simulink model "vehicle_motion_model_final_temp"  (R2021b)
settings: Solver=ode5  StartTime=0.0  StopTime=600  FixedStep=0.001  RelTol=1e-3
StopFcn:
  | % stop simulation callback function
  | figure(1);
  | out.x_gt.data = permute(out.x_gt.data,[3, 1, 2]);
  | plot3(out.x_gt.data(:, 1), out.x_gt.data(:, 2), -out.x_gt.data(:, 3), 'Color', 'r', 'LineWidth', 1.5);
  | legend('Истинная траектория')
  | xlabel('X, \itм');
  | ylabel('Y, \itм');
  | zlabel('Z, \itм');
  | figure(2);
  | plot3(out.x.data(:, 1), out.x.data(:, 2), -out.x.data(:, 3), 'Color', 'b', 'LineWidth', 1.5);
  | hold on;
  | xlabel('X, \itм');
  | ylabel('Y, \itм');
  | zlabel('Z, \itм');
  | % legend('pos')
  | hold on;
  | plot3(out.x_gt.data(:, 1), out.x_gt.data(:, 2), -out.x_gt.data(:, 3), 'Color', 'r', 'LineWidth', 1.5);
  | hold on;
  | legend('Рассчитанная траектория', 'Истинная траектория')
  | % errors
  | figure(3);
  | yyaxis left;
  | plot(out.hor_err_fus.time, out.hor_err_fus.data, 'Color', 'b', 'LineWidth', 1.5);
  | xlabel('время, \itс');
  | ylabel('Горизонтальная ошибка, \itм');
  | hold on;
  | yyaxis right;
  | plot(out.ver_err_fus.time, out.ver_err_fus.data, 'Color', 'r', 'LineWidth', 1.5);
  | ylabel('Вертикальная ошибка, \itм');
  | legend('Горизонтальная позиционная ошибка', 'Вертикальная позиционная ошибка');
  | grid on;
  | figure(4);
  | yyaxis left;
  | plot(out.hor_err_ins.time, out.hor_err_ins.data, '-', 'Color', 'b', 'LineWidth', 1.5);
  | xlabel('время, \itс');
  | ylabel('Горизонтальная ошибка, \itм');
  | hold on;
  | yyaxis right;
  | plot(out.ver_err_ins.time, out.ver_err_ins.data, '-', 'Color', 'r', 'LineWidth', 1.5);
  | ylabel('Вертикальная ошибка, \itм');
  | legend('Горизонтальная позиционная ошибка', 'Вертикальная позиционная ошибка');
  | grid on;
model workspace (MAT data in the model file):
  AxlIxx = 62.3745166667
  AxlM = 160
  Cps = 2
  CzWhlAxl = 557955.087061
  DCT_Param : object (value not decoded)
  Downshift_Speeds = [9.5625 12.9375 16.3125 19.6875 23.0625 26.4375 29.8125 33.1875 36.5625 39.9375 43.3125 46.6875 ... (28 elements, 4x7)]
  F0zWhlAxl = 16132.2380068
  HTCH : object (value not decoded)
  Hmax = 0.25
  KzWhlAxl = 58428920.0848
  NCyl = 6
  Pedal_Positions = [0.1 0.4 0.5 0.9]
  Pstd = 101325
  Q = [1  0  0; 0  1  0; 0  0  1]
  Rair = 287
  SUS : object (value not decoded)
  TRA : object (value not decoded)
  Trans : object (value not decoded)
  Tstd = 293.15
  Upshift_Speeds = [12.9375 16.3125 19.6875 33 26.4375 29.8125 33.1875 52.5 39.9375 43.3125 46.6875 77.25 ... (28 elements, 4x7)]
  VEH : object (value not decoded)
  Vd = 0.00346
  WH : Mass (value not decoded)
  dt3D = 0.05
  f_air = [0 0 0 0 0 0 0 0 0 0 0 0 ... (256 elements, 16x16)]
  f_co = [0 0 0 0 0 0 0 0 0 0 0 0 ... (256 elements, 16x16)]
  f_co2 = [0 0 0 0 0 0 0 0 0 0 0 0 ... (256 elements, 16x16)]
  f_eff = [352.135682859 352.135682859 320.724378192 303.655312657 295.930136708 291.240087194 291.240271258 291.240312459 291.240275452 291.240198499 291.240100781 291.240018769 ... (256 elements, 16x16)]
  f_fuel = [0 0 0 0 0 0 0 0 0 0 0 0 ... (256 elements, 16x16)]
  f_hc = [0 0 0 0 0 0 0 0 0 0 0 0 ... (256 elements, 16x16)]
  f_nox = [0 0 0 0 0 0 0 0 0 0 0 0 ... (256 elements, 16x16)]
  f_pm = [0 0 0 0 0 0 0 0 0 0 0 0 ... (256 elements, 16x16)]
  f_susp_axl_bp = [1 2]
  f_susp_dz_bp = [-0.325022776267 -0.315022776267 -0.305022776267 -0.205022776267 -0.105022776267 -0.00502277626717 0.0949772237328 0.194977223733 0.204977223733 0.214977223733]
  f_susp_dzdot_bp = [-3 -0.3 -0.2 -0.1 0 0.1 0.2 0.3 3]
  f_susp_fmz = [-144070.391448 -93629.24037 -75929.1118915 -20630.5828179 -15385.48216 -10140.3815021 -4895.28084414 349.819813785 -31916.3973792 18437.6709544 -83996.1993354 -33555.0482577 ... (43920 elements, 10x9x61x2x4)]
  f_susp_geom = [0 0 0 0 0 0 0 0 0 0 0 0 ... (3660 elements, 10x61x2x3)]
  f_susp_strgdelta_bp = [-0.523598775598 -0.506145483078 -0.488692190558 -0.471238898038 -0.453785605519 -0.436332312999 -0.418879020479 -0.401425727959 -0.383972435439 -0.366519142919 -0.349065850399 -0.331612557879 ... (61 elements, 1x61)]
  f_tbrake = [0 76.8593923996 105.140482948 131.533638111 157.926793274 176.658631717 176.65727296 176.656856686 176.656879077 176.657093756 176.657404516 176.65772406 ... (256 elements, 16x16)]
  f_tbrake_n_bpt = [0 649.519052838 912.419621844 1175.32019085 1438.22075986 1701.12132886 1964.02189787 2226.92246687 2489.82303588 2752.72360489 3015.62417389 3278.5247429 ... (16 elements, 1x16)]
  f_tbrake_t_bpt = [0 34.6410161514 61.0341713143 87.4273264773 113.82048164 140.213636803 166.606791966 192.999947129 219.393102292 245.786257455 272.179412618 298.572567781 ... (16 elements, 1x16)]
  f_texh = [766.752464599 766.752464599 786.17542386 801.679939032 884.591982581 910.574397722 910.571871054 910.570774534 910.570601632 910.570821151 910.571247242 910.571639815 ... (256 elements, 16x16)]
  f_twc_eff_co = [0.17 0.25 0.45 0.99 0.99 0.99 0.99]
  f_twc_eff_hc = [0.21 0.375 0.75 0.98 0.98 0.98 0.98]
  f_twc_eff_lam = [0.909090909 0.944055944 0.979020979 1 1.013986014 1.048951049 1.083916084]
  f_twc_eff_nox = [0.98 0.98 0.98 0.97 0.05 0.02 0]
  h = 0.134
symbols that are objects in the model workspace (value not decoded): VEH
libraries: aerolibcommonsys x8, sharedtransform x8, sharedutil x7, autolibsharedcommon x7, autolibutils x4, vehdynlibtirecommon x3, dspstat3 x2, mspsensorlib x1, aerolibnav x1, shared6dof x1, autolibshared x1, vehdynlibsuspension x1
(part 7 of 9)

== system vehicle_motion_model_final_temp/Two-Axle Vehicle/Wheels and Tires/Wheels and Tires/Tires/MF Tires ==
  DriveTorque : Inport
  Brake Pressure : Inport  Port=2
  r : Inport  Port=3
  Vx : Inport  Port=4
  Vy : Inport  Port=5
  Camber : Inport  Port=6
  Press : Inport  Port=7  Unit=Pa
  lambda : Inport  Port=8  Unit=1
  Gnd : Inport  Port=9
  FzSusp : Inport  Port=10
  Combined Slip Wheel 2DOF : Subsystem  AncestorBlock=vehdynlibtire/Combined Slip Wheel 2DOF  mask(Combined Slip Wheel 2DOF){tireType=Commercial truck 295/75R22.5, BrakeType=Disc, plySteer=off, turnslip=off, mu_static=.3, mu_kinetic=.2, disk_abore=.05, Rm=.177, num_pads=2, drum_abore=0.0508, drum_a=0.123, drum_c=0.212, drum_r=0.15, drum_theta1=0, drum_theta2=126, brake_p_bpt=[1 11.4736842105263 21.9473684210526 32.4210526315789 42.8947368421053 53.3684210526316 63.8421052631579 74.3157894736842 84.7894736842105 95.2631578947368 105.736842105263 116.210526315789 126.684210526316 137.157894736842 147.631578947368 158.105263157895 168.578947368421 179.052631578947 189.526315789474 200], brake_n_bpt=[0 52.6315789473684 105.263157894737 157.894736842105 210.526315789474 263.157894736842 315.789473684211 368.421052631579 421.052631578947 473.684210526316 526.315789473684 578.947368421053 631.578947368421 684.210526315789 736.842105263158 789.473684210526 842.105263157895 894.736842105263 947.368421052632 1000], f_brake_t=[43.4900602404453 42.5056030554862 41.5350898940194 40.5780454442085 39.6340111501808 38.7025443887544 37.7832176914519 36.8756180088306 35.9793460143796 35.0940154454303 34.2192524787115 33.3546951383474 32.4999927342521 31.6548053290159 30.8188032315107 29.991666515561 29.1730845621415 28.362755623661 27.5603864089927 26.765691687993;498.991217495636 487.695866636631 476.560505099801 465.579679307235 454.748127933653 444.060772460445 433.51270824929 423.099196101319 412.81565427025 402.657650900201 392.620896861006 382.701238955775 372.894653477208 363.197240090814 353.605216024701 344.114910546964 334.722759712992 325.425301366216 316.219170376863 307.10109410434;954.492374750826 932.886130217776 911.585920305583 890.581313170261 869.862244717126 849.419000532136 829.242198807128 809.322774193808 789.651962526121 770.221286354971 751.0225412433 732.047782773203 713.289314220164 694.739674852612 676.391628817892 658.238154578366 640.272434863842 622.48784710877 604.877954344734 587.436496520688;1409.99353200602 1378.07639379892 1346.61133551136 1315.58294703329 1284.9763615006 1254.77722860383 1224.97168936497 1195.5463522863 1166.48827078199 1137.78492180974 1109.42418562559 1081.39432659063 1053.68397496312 1026.28210961441 999.178041611083 972.361398609768 945.822110014692 919.550392851325 893.536738312604 867.771898937035;1865.49468926121 1823.26665738007 1781.63675071715 1740.58458089631 1700.09047828407 1660.13545667552 1620.7011799228 1581.76993037878 1543.32457903786 1505.34855726451 1467.82583000789 1430.74087040806 1394.07863570608 1357.82454437621 1321.96445440427 1286.48464264117 1251.37178516554 1216.61293859388 1182.19552228048 1148.10730135338;2320.9958465164 2268.45692096121 2216.66216592293 2165.58621475934 2115.20459506754 2065.49368474721 2016.43067048064 1967.99350847127 1920.16088729373 1872.91219271928 1826.22747439018 1780.08741422549 1734.47329644903 1689.36697913801 1644.75086719747 1600.60788667257 1556.92146031639 1513.67548433643 1470.85430624835 1428.44270376973;2776.49700377159 2713.64718454235 2651.68758112871 2590.58784862237 2530.31871185102 2470.8519128189 2412.16016103848 2354.21708656376 2296.9971955496 2240.47582817405 2184.62911877248 2129.43395804292 2074.86795719199 2020.9094138998 1967.53727999066 1914.73113070398 1862.47113546724 1810.73803007899 1759.51309021622 1708.77810618608;3231.99816102678 3158.8374481235 3086.71299633449 3015.58948248539 2945.43282863449 2876.21014089059 2807.88965159632 2740.44066465625 2673.83350380547 2608.03946362882 2543.03076315477 2478.78050186034 2415.26261793494 2352.4518486616 2290.32369278385 2228.85437473538 2168.02081061809 2107.80057582154 2048.17187418409 1989.11350860242;3687.49931828197 3604.02771170464 3521.73841154027 3440.59111634842 3360.54694541796 3281.56836896228 3203.61914215416 3126.66424274874 3050.66981206134 2975.60309908359 2901.43240753707 2828.12704567777 2755.6572786779 2683.9942834234 2613.11010557704 2542.97761876678 2473.57048576894 2404.8631215641 2336.83065815196 2269.44891101877;4143.00047553716 4049.21797528579 3956.76382674606 3865.59275021144 3775.66106220143 3686.92659703397 3599.34863271199 3512.88782084123 3427.50612031721 3343.16673453836 3259.83405191936 3177.4735894952 3096.05193942085 3015.5367181852 2935.89651837023 2857.10086279818 2779.12016091979 2701.92566730665 2625.48944211983 2549.78431343512;4598.50163279235 4494.40823886693 4391.78924195184 4290.59438407447 4190.77517898491 4092.28482510566 3995.07812326983 3899.11139893372 3804.34242857308 3710.73036999313 3618.23569630166 3526.82013331263 3436.44660016381 3347.079152947 3258.68293116342 3171.22410682959 3084.66983607064 2998.98821304921 2914.1482260877 2830.11971585147;5054.00279004754 4939.59850244808 4826.81465715762 4715.59601793749 4605.88929576838 4497.64305317735 4390.80761382767 4285.3349770262 4181.17873682896 4078.2940054479 3976.63734068395 3876.16667713006 3776.84126090677 3678.62158770879 3581.46934395661 3485.34735086099 ...(+2764 chars)], tireParamSet=vdynPassCar.mat, PRESMAX=1000000, PRESMIN=10000, FZMAX=28000, FZMIN=100, VXLOW=1, KPUMAX=1.5, KPUMIN=-1.5, ALPMAX=1.5, ALPMIN=-1.5, CAMMAX=0.17453, CAMMIN=-0.17453, LONGVL=16.7, FxRelFreqLwrLim=200*pi, FyRelFreqLwrLim=200*pi, MyRelFreqLwrLim=100*pi, omegao=0, br=1e-3, UNLOADED_RADIUS=0.5132, NOMPRES=793000, FNOMIN=14000, WIDTH=0.295, RIM_RADIUS=0.28575, MASS=54.96, IYY=10.664, GRAVITY=-9.81, zo=.015+VEH.InitialVertPosition, zdoto=0, BREFF=8.25094594147963, DREFF=0.260468730454265, FREFF=0.0735298544471851, Q_RE0=1.00866439868088, Q_V1=0.000760413786224011, Q_V2=0.0463384792019201, Q_FZ1=0, Q_FZ2=15.6870832810226, Q_FZ3=0, Q_FCX=0.138643970247602, Q_FCY=0.10843499565426, Q_FCY2=-0.465763352339538, PFZ1=0.69958166705601, VERTICAL_STIFFNESS=207885.061134007, VERTICAL_DAMPING=1000, BOTTOM_OFFST=.01, BOTTOM_STIFF=2e6, LONGITUDINAL_STIFFNESS=388714.175879854, LATERAL_STIFFNESS=157087.404633332, PCFX1=0.18539229191199, PCFX2=0, PCFX3=0, PCFY1=0.163183345037677, PCFY2=0, PCFY3=0.249094918231954, Q_RA1=0.675942571700787, Q_RA2=0.73800463546164, Q_RB1=1.04487486456705, Q_RB2=-1.191763806629, PCX1=1.58523057950359, PDX1=1.0239116238178, PDX2=-0.0842405110022724, PDX3=0, PEX1=0.110312777158455, PEX2=0.313468516038146, PEX3=0, PEX4=0.0016060905760045, PKX1=21.3872544684023, PKX2=14.0006541873175, PKX3=-0.405326109653452, PHX1=0.000212599305364818, PHX2=0.00115950515263055, PVX1=1.59236164471432e-05, PVX2=0.000104321112127671, PPX1=-0.349461321276586, PPX2=0.387840040616429, PPX3=-0.0969947336569324, PPX4=0.0632271859795801, RBX1=12.7633329850276, RBX2=9.5787123658471, RBX3=0, RCX1=1.02796280922059, REX1=-0.45202516851367, REX2=-0.47304886171176, RHX1=0.000233272373115809, QSX1=-0.00788307788961443, QSX2=0.954629515459396, QSX3=0.0155855777667025, QSX4=0.125904607142414, QSX5=1.01110069703963, QSX6=20.1938577118433, QSX7=0.310818120717083, QSX8=-0.0430823751139655, QSX9=0.636494404888216, QSX10=0.142438060591663, QSX11=0.346766530036373, QSX12=0, QSX13=0, QSX14=0, PPMX1=0, PCY1=1.34299950037631, PDY1=0.878267729082195, PDY2=-0.0644597923147385, PDY3=0, PEY1=-0.809776534470972, PEY2=-0.600180598867198, PEY3=0.0991732552633487, PEY4=-6.5577974035573, PEY5=0, PKY1=-15.5714726518315, PKY2=1.73126522291751, PKY3=0.365349873517229, PKY4=1.98176755955416, PKY5=0, PKY6=-0.884005199550313, PKY7=-0.237259727611847, PHY1=-0.00183370557235628, PHY2=0.00346401302716671, PVY1=-0.00675427560163264, PVY2=0.036379218103843, PVY3=-0.163543984089166, PVY4=-0.491003349625726, PPY1=-0.62059646553185, PPY2=-0.0647824842338686, PPY3=-0.164648843290686, PPY4=0.283193909060098, PPY5=0, RBY1=10.7588809173639, RBY2=7.70420065295029, RBY3=3.40283755070691e-06, RBY4=0, RCY1=1.06691874059059, REY1=0.308244924574305, REY2=7.48775032604508e-06, RHY1=0.0118479204960415, RHY2=7.63650177161071e-06, RVY1=0.0560024425050078, RVY2=7.48487127056197e-06, RVY3=0, RVY4=98.4047026517149, RVY5=2.02759273900054, RVY6=15.7623064923347, QSY1=0.00699077564863536, QSY2=0, QSY3=0.00153535478298811, QSY4=8.55710322455322e-05, QSY5=0, QSY6=0, QSY7=0.89443879773793, QSY8=-0.403227641260894, QBZ1=11.666656027484, QBZ2=-1.30355438574485, QBZ3=0, QBZ4=0.177918305399071, QBZ5=-0.162481135068033, QBZ6=0, QBZ9=30.1445534682089, QBZ10=0, QCZ1=1.29026978207574, QDZ1=0.0886972644991399, QDZ2=-0.0058634820161856, QDZ3=0.3805597481383, QDZ4=0, QDZ6=0.00160914918118959, QDZ7=-0.00211036330862154, QDZ8=-0.13921904912557, QDZ9=0.00816585550028243, QDZ10=0, QDZ11=0, QEZ1=-2.19802254534746, QEZ2=1.01850535789165, QEZ3=0, QEZ4=0.278379679112054, QEZ5=-0.548414722765386, QHZ1=0.00148361198869669, QHZ2=0.00202017567585904, QHZ3=0.240316641332066, QHZ4=-0.210114035738085, PPZ1=-0.443927982388615, PPZ2=0, SSZ1=0.00914999585397887, SSZ2=0.0389830656052735, SSZ3=0, SSZ4=0, PDXP1=0.396718274678791, PDXP2=0, PDXP3=0, PKYP1=1.00587060633573, PDYP1=0.40483048923438, PDYP2=0, PDYP3=0, PDYP4=0, PHYP1=0.992731942067188, PHYP2=0.150352945499914, PHYP3=0, PHYP4=-3.98988682633674, PECP1=0.502379254513503, PECP2=0, QDTP1=10.0178654287947, QCRP1=0.200627747200702, QCRP2=0.0995735881599772, QBRP1=0.0997107127960717, QDRP1=1.01432910167423, QDRP2=0, aMode=2}
      mask prompts: tireType "vdynblks:vehdynLatTire:blkPrm_tireType"; BrakeType "vdynblks:vehdynLatTire:blkPrm_BrakeType"; plySteer "vdynblks:vehdynLatTire:blkPrm_plySteer"; turnslip "vdynblks:vehdynLatTire:blkPrm_turnslip"; mu_static "autoblks_shared:autoblkLongitudinalWheel:blkPrm_mu_static"; mu_kinetic "autoblks_shared:autoblkLongitudinalWheel:blkPrm_mu_kinetic"; disk_abore "autoblks_shared:autoblkLongitudinalWheel:blkPrm_disk_abore"; Rm "autoblks_shared:autoblkLongitudinalWheel:blkPrm_Rm"; num_pads "autoblks_shared:autoblkLongitudinalWheel:blkPrm_num_pads"; drum_abore "autoblks_shared:autoblkLongitudinalWheel:blkPrm_drum_abore"; drum_a "autoblks_shared:autoblkLongitudinalWheel:blkPrm_drum_a"; drum_c "autoblks_shared:autoblkLongitudinalWheel:blkPrm_drum_c"; drum_r "autoblks_shared:autoblkLongitudinalWheel:blkPrm_drum_r"; drum_theta1 "autoblks_shared:autoblkLongitudinalWheel:blkPrm_drum_theta1"; drum_theta2 "autoblks_shared:autoblkLongitudinalWheel:blkPrm_drum_theta2"; brake_p_bpt "autoblks_shared:autoblkLongitudinalWheel:blkPrm_brake_p_bpt"; brake_n_bpt "autoblks_shared:autoblkLongitudinalWheel:blkPrm_brake_n_bpt"; f_brake_t "autoblks_shared:autoblkLongitudinalWheel:blkPrm_f_brake_t"; tireParamSet "vdynblks:vehdynLatTire:blkPrm_tireParamSet"; PRESMAX "vdynblks:vehdynLatTire:blkPrm_PRESMAX"; PRESMIN "vdynblks:vehdynLatTire:blkPrm_PRESMIN"; FZMAX "vdynblks:vehdynLatTire:blkPrm_FZMAX"; FZMIN "vdynblks:vehdynLatTire:blkPrm_FZMIN"; VXLOW "vdynblks:vehdynLatTire:blkPrm_VXLOW"; KPUMAX "vdynblks:vehdynLatTire:blkPrm_KPUMAX"; KPUMIN "vdynblks:vehdynLatTire:blkPrm_KPUMIN"; ALPMAX "vdynblks:vehdynLatTire:blkPrm_ALPMAX"; ALPMIN "vdynblks:vehdynLatTire:blkPrm_ALPMIN"; CAMMAX "vdynblks:vehdynLatTire:blkPrm_CAMMAX"; CAMMIN "vdynblks:vehdynLatTire:blkPrm_CAMMIN"; LONGVL "vdynblks:vehdynLatTire:blkPrm_LONGVL"; FxRelFreqLwrLim "Longitudinal relaxation length lower frequency limit, FxRelFreqLwrLim [rad/s]:"; FyRelFreqLwrLim "Lateral relaxation length lower frequency limit, FyRelFreqLwrLim [rad/s]:"; MyRelFreqLwrLim "Rolling relaxation length lower frequency limit, MyRelFreqLwrLim [rad/s]:"; omegao "vdynblks:vehdynLatTire:blkPrm_omegao"; br "vdynblks:vehdynLatTire:blkPrm_br"; UNLOADED_RADIUS "vdynblks:vehdynLatTire:blkPrm_UNLOADED_RADIUS"; NOMPRES "vdynblks:vehdynLatTire:blkPrm_NOMPRES"; FNOMIN "vdynblks:vehdynLatTire:blkPrm_FNOMIN"; WIDTH "vdynblks:vehdynLatTire:blkPrm_WIDTH"; RIM_RADIUS "vdynblks:vehdynLatTire:blkPrm_RIM_RADIUS"; MASS "vdynblks:vehdynLatTire:blkPrm_MASS"; IYY "vdynblks:vehdynLatTire:blkPrm_IYY"; GRAVITY "vdynblks:vehdynLatTire:blkPrm_GRAVITY"; zo "vdynblks:vehdynLatTire:blkPrm_zo"; zdoto "vdynblks:vehdynLatTire:blkPrm_zdoto"; BREFF "vdynblks:vehdynLatTire:blkPrm_BREFF"; DREFF "vdynblks:vehdynLatTire:blkPrm_DREFF"; FREFF "vdynblks:vehdynLatTire:blkPrm_FREFF"; Q_RE0 "vdynblks:vehdynLatTire:blkPrm_Q_RE0"; Q_V1 "vdynblks:vehdynLatTire:blkPrm_Q_V1"; Q_V2 "vdynblks:vehdynLatTire:blkPrm_Q_V2"; Q_FZ1 "vdynblks:vehdynLatTire:blkPrm_Q_FZ1"; Q_FZ2 "vdynblks:vehdynLatTire:blkPrm_Q_FZ2"; Q_FZ3 "vdynblks:vehdynLatTire:blkPrm_Q_FZ3"; Q_FCX "vdynblks:vehdynLatTire:blkPrm_Q_FCX"; Q_FCY "vdynblks:vehdynLatTire:blkPrm_Q_FCY"; Q_FCY2 "vdynblks:vehdynLatTire:blkPrm_Q_FCY2"; PFZ1 "vdynblks:vehdynLatTire:blkPrm_PFZ1"; VERTICAL_STIFFNESS "vdynblks:vehdynLatTire:blkPrm_VERTICAL_STIFFNESS"; VERTICAL_DAMPING "vdynblks:vehdynLatTire:blkPrm_VERTICAL_DAMPING"; BOTTOM_OFFST "vdynblks:vehdynLatTire:blkPrm_BOTTOM_OFFST"; BOTTOM_STIFF "vdynblks:vehdynLatTire:blkPrm_BOTTOM_STIFF"; LONGITUDINAL_STIFFNESS "vdynblks:vehdynLatTire:blkPrm_LONGITUDINAL_STIFFNESS"; LATERAL_STIFFNESS "vdynblks:vehdynLatTire:blkPrm_LATERAL_STIFFNESS"; PCFX1 "vdynblks:vehdynLatTire:blkPrm_PCFX1"; PCFX2 "vdynblks:vehdynLatTire:blkPrm_PCFX2"; PCFX3 "vdynblks:vehdynLatTire:blkPrm_PCFX3"; PCFY1 "vdynblks:vehdynLatTire:blkPrm_PCFY1"; PCFY2 "vdynblks:vehdynLatTire:blkPrm_PCFY2"; PCFY3 "vdynblks:vehdynLatTire:blkPrm_PCFY3"; Q_RA1 "vdynblks:vehdynLatTire:blkPrm_Q_RA1"; Q_RA2 "vdynblks:vehdynLatTire:blkPrm_Q_RA2"; Q_RB1 "vdynblks:vehdynLatTire:blkPrm_Q_RB1"; Q_RB2 "vdynblks:vehdynLatTire:blkPrm_Q_RB2"; PCX1 "vdynblks:vehdynLatTire:blkPrm_PCX1"; PDX1 "vdynblks:vehdynLatTire:blkPrm_PDX1"; PDX2 "vdynblks:vehdynLatTire:blkPrm_PDX2"; PDX3 "vdynblks:vehdynLatTire:blkPrm_PDX3"; PEX1 "vdynblks:vehdynLatTire:blkPrm_PEX1"; PEX2 "vdynblks:vehdynLatTire:blkPrm_PEX2"; PEX3 "vdynblks:vehdynLatTire:blkPrm_PEX3"; PEX4 "vdynblks:vehdynLatTire:blkPrm_PEX4"; PKX1 "vdynblks:vehdynLatTire:blkPrm_PKX1"; PKX2 "vdynblks:vehdynLatTire:blkPrm_PKX2"; PKX3 "vdynblks:vehdynLatTire:blkPrm_PKX3"; PHX1 "vdynblks:vehdynLatTire:blkPrm_PHX1"; PHX2 "vdynblks:vehdynLatTire:blkPrm_PHX2"; PVX1 "vdynblks:vehdynLatTire:blkPrm_PVX1"; PVX2 "vdynblks:vehdynLatTire:blkPrm_PVX2"; PPX1 "vdynblks:vehdynLatTire:blkPrm_PPX1"; PPX2 "vdynblks:vehdynLatTire:blkPrm_PPX2"; PPX3 "vdynblks:vehdynLatTire:blkPrm_PPX3"; PPX4 "vdynblks:vehdynLatTire:blkPrm_PPX4"; RBX1 "vdynblks:vehdynLatTire:blkPrm_RBX1"; RBX2 "vdynblks:vehdynLatTire:blkPrm_RBX2"; RBX3 "vdynblks:vehdynLatTire:blkPrm_RBX3"; RCX1 "vdynblks:vehdynLatTire:blkPrm_RCX1"; REX1 "vdynblks:vehdynLatTire:blkPrm_REX1"; REX2 "vdynblks:vehdynLatTire:blkPrm_REX2"; RHX1 "vdynblks:vehdynLatTire:blkPrm_RHX1"; QSX1 "vdynblks:vehdynLatTire:blkPrm_QSX1"; QSX2 "vdynblks:vehdynLatTire:blkPrm_QSX2"; QSX3 "vdynblks:vehdynLatTire:blkPrm_QSX3"; QSX4 "vdynblks:vehdynLatTire:blkPrm_QSX4"; QSX5 "vdynblks:vehdynLatTire:blkPrm_QSX5"; QSX6 "vdynblks:vehdynLatTire:blkPrm_QSX6"; QSX7 "vdynblks:vehdynLatTire:blkPrm_QSX7"; QSX8 "vdynblks:vehdynLatTire:blkPrm_QSX8"; QSX9 "vdynblks:vehdynLatTire:blkPrm_QSX9"; QSX10 "vdynblks:vehdynLatTire:blkPrm_QSX10"; QSX11 "vdynblks:vehdynLatTire:blkPrm_QSX11"; QSX12 "vdynblks:vehdynLatTire:blkPrm_QSX12"; QSX13 "vdynblks:vehdynLatTire:blkPrm_QSX13"; QSX14 "vdynblks:vehdynLatTire:blkPrm_QSX14"; PPMX1 "vdynblks:vehdynLatTire:blkPrm_PPMX1"; PCY1 "vdynblks:vehdynLatTire:blkPrm_PCY1"; PDY1 "vdynblks:vehdynLatTire:blkPrm_PDY1"; PDY2 "vdynblks:vehdynLatTire:blkPrm_PDY2"; PDY3 "vdynblks:vehdynLatTire:blkPrm_PDY3"; PEY1 "vdynblks:vehdynLatTire:blkPrm_PEY1"; PEY2 "vdynblks:vehdynLatTire:blkPrm_PEY2"; PEY3 "vdynblks:vehdynLatTire:blkPrm_PEY3"; PEY4 "vdynblks:vehdynLatTire:blkPrm_PEY4"; PEY5 "vdynblks:vehdynLatTire:blkPrm_PEY5"; PKY1 "vdynblks:vehdynLatTire:blkPrm_PKY1"; PKY2 "vdynblks:vehdynLatTire:blkPrm_PKY2"; PKY3 "vdynblks:vehdynLatTire:blkPrm_PKY3"; PKY4 "vdynblks:vehdynLatTire:blkPrm_PKY4"; PKY5 "vdynblks:vehdynLatTire:blkPrm_PKY5"; PKY6 "vdynblks:vehdynLatTire:blkPrm_PKY6"; PKY7 "vdynblks:vehdynLatTire:blkPrm_PKY7"; PHY1 "vdynblks:vehdynLatTire:blkPrm_PHY1"; PHY2 "vdynblks:vehdynLatTire:blkPrm_PHY2"; PVY1 "vdynblks:vehdynLatTire:blkPrm_PVY1"; PVY2 "vdynblks:vehdynLatTire:blkPrm_PVY2"; PVY3 "vdynblks:vehdynLatTire:blkPrm_PVY3"; PVY4 "vdynblks:vehdynLatTire:blkPrm_PVY4"; PPY1 "vdynblks:vehdynLatTire:blkPrm_PPY1"; PPY2 "vdynblks:vehdynLatTire:blkPrm_PPY2"; PPY3 "vdynblks:vehdynLatTire:blkPrm_PPY3"; PPY4 "vdynblks:vehdynLatTire:blkPrm_PPY4"; PPY5 "vdynblks:vehdynLatTire:blkPrm_PPY5"; RBY1 "vdynblks:vehdynLatTire:blkPrm_RBY1"; RBY2 "vdynblks:vehdynLatTire:blkPrm_RBY2"; RBY3 "vdynblks:vehdynLatTire:blkPrm_RBY3"; RBY4 "vdynblks:vehdynLatTire:blkPrm_RBY4"; RCY1 "vdynblks:vehdynLatTire:blkPrm_RCY1"; REY1 "vdynblks:vehdynLatTire:blkPrm_REY1"; REY2 "vdynblks:vehdynLatTire:blkPrm_REY2"; RHY1 "vdynblks:vehdynLatTire:blkPrm_RHY1"; RHY2 "vdynblks:vehdynLatTire:blkPrm_RHY2"; RVY1 "vdynblks:vehdynLatTire:blkPrm_RVY1"; RVY2 "vdynblks:vehdynLatTire:blkPrm_RVY2"; RVY3 "vdynblks:vehdynLatTire:blkPrm_RVY3"; RVY4 "vdynblks:vehdynLatTire:blkPrm_RVY4"; RVY5 "vdynblks:vehdynLatTire:blkPrm_RVY5"; RVY6 "vdynblks:vehdynLatTire:blkPrm_RVY6"; QSY1 "vdynblks:vehdynLatTire:blkPrm_QSY1"; QSY2 "vdynblks:vehdynLatTire:blkPrm_QSY2"; QSY3 "vdynblks:vehdynLatTire:blkPrm_QSY3"; QSY4 "vdynblks:vehdynLatTire:blkPrm_QSY4"; QSY5 "vdynblks:vehdynLatTire:blkPrm_QSY5"; QSY6 "vdynblks:vehdynLatTire:blkPrm_QSY6"; QSY7 "vdynblks:vehdynLatTire:blkPrm_QSY7"; QSY8 "vdynblks:vehdynLatTire:blkPrm_QSY8"; QBZ1 "vdynblks:vehdynLatTire:blkPrm_QBZ1"; QBZ2 "vdynblks:vehdynLatTire:blkPrm_QBZ2"; QBZ3 "vdynblks:vehdynLatTire:blkPrm_QBZ3"; QBZ4 "vdynblks:vehdynLatTire:blkPrm_QBZ4"; QBZ5 "vdynblks:vehdynLatTire:blkPrm_QBZ5"; QBZ6 "vdynblks:vehdynLatTire:blkPrm_QBZ6"; QBZ9 "vdynblks:vehdynLatTire:blkPrm_QBZ9"; QBZ10 "vdynblks:vehdynLatTire:blkPrm_QBZ10"; QCZ1 "vdynblks:vehdynLatTire:blkPrm_QCZ1"; QDZ1 "vdynblks:vehdynLatTire:blkPrm_QDZ1"; QDZ2 "vdynblks:vehdynLatTire:blkPrm_QDZ2"; QDZ3 "vdynblks:vehdynLatTire:blkPrm_QDZ3"; QDZ4 "vdynblks:vehdynLatTire:blkPrm_QDZ4"; QDZ6 "vdynblks:vehdynLatTire:blkPrm_QDZ6"; QDZ7 "vdynblks:vehdynLatTire:blkPrm_QDZ7"; QDZ8 "vdynblks:vehdynLatTire:blkPrm_QDZ8"; QDZ9 "vdynblks:vehdynLatTire:blkPrm_QDZ9"; QDZ10 "vdynblks:vehdynLatTire:blkPrm_QDZ10"; QDZ11 "vdynblks:vehdynLatTire:blkPrm_QDZ11"; QEZ1 "vdynblks:vehdynLatTire:blkPrm_QEZ1"; QEZ2 "vdynblks:vehdynLatTire:blkPrm_QEZ2"; QEZ3 "vdynblks:vehdynLatTire:blkPrm_QEZ3"; QEZ4 "vdynblks:vehdynLatTire:blkPrm_QEZ4"; QEZ5 "vdynblks:vehdynLatTire:blkPrm_QEZ5"; QHZ1 "vdynblks:vehdynLatTire:blkPrm_QHZ1"; QHZ2 "vdynblks:vehdynLatTire:blkPrm_QHZ2"; QHZ3 "vdynblks:vehdynLatTire:blkPrm_QHZ3"; QHZ4 "vdynblks:vehdynLatTire:blkPrm_QHZ4"; PPZ1 "vdynblks:vehdynLatTire:blkPrm_PPZ1"; PPZ2 "vdynblks:vehdynLatTire:blkPrm_PPZ2"; SSZ1 "vdynblks:vehdynLatTire:blkPrm_SSZ1"; SSZ2 "vdynblks:vehdynLatTire:blkPrm_SSZ2"; SSZ3 "vdynblks:vehdynLatTire:blkPrm_SSZ3"; SSZ4 "vdynblks:vehdynLatTire:blkPrm_SSZ4"; PDXP1 "vdynblks:vehdynLatTire:blkPrm_PDXP1"; PDXP2 "vdynblks:vehdynLatTire:blkPrm_PDXP2"; PDXP3 "vdynblks:vehdynLatTire:blkPrm_PDXP3"; PKYP1 "vdynblks:vehdynLatTire:blkPrm_PKYP1"; PDYP1 "vdynblks:vehdynLatTire:blkPrm_PDYP1"; PDYP2 "vdynblks:vehdynLatTire:blkPrm_PDYP2"; PDYP3 "vdynblks:vehdynLatTire:blkPrm_PDYP3"; PDYP4 "vdynblks:vehdynLatTire:blkPrm_PDYP4"; PHYP1 "vdynblks:vehdynLatTire:blkPrm_PHYP1"; PHYP2 "vdynblks:vehdynLatTire:blkPrm_PHYP2"; PHYP3 "vdynblks:vehdynLatTire:blkPrm_PHYP3"; PHYP4 "vdynblks:vehdynLatTire:blkPrm_PHYP4"; PECP1 "vdynblks:vehdynLatTire:blkPrm_PECP1"; PECP2 "vdynblks:vehdynLatTire:blkPrm_PECP2"; QDTP1 "vdynblks:vehdynLatTire:blkPrm_QDTP1"; QCRP1 "vdynblks:vehdynLatTire:blkPrm_QCRP1"; QCRP2 "vdynblks:vehdynLatTire:blkPrm_QCRP2"; QBRP1 "vdynblks:vehdynLatTire:blkPrm_QBRP1"; QDRP1 "vdynblks:vehdynLatTire:blkPrm_QDRP1"; QDRP2 "vdynblks:vehdynLatTire:blkPrm_QDRP2"
      mask help: vdynblks:vehdynLatTire:blkDesc
      mask init:
      | vdynMF=vehdynicon('vehdynlibtire',gcb,0);
      mask Help: eval('vdynblkshelp(''vbtireslip'')')
      mask TypeOptions tireType: vdynblks:vehdynLatTire:blkCmb_tireType_c1 | vdynblks:vehdynLatTire:blkCmb_tireType_c2 | vdynblks:vehdynLatTire:blkCmb_tireType_c3 | vdynblks:vehdynLatTire:blkCmb_tireType_c4 | vdynblks:vehdynLatTire:blkCmb_tireType_c5 | vdynblks:vehdynLatTire:blkCmb_tireType_c6 | vdynblks:vehdynLatTire:blkCmb_tireType_c7
      mask Callback tireType: [~]=vehdynicon('vehdynlibtire',gcb,5)
      mask TypeOptions BrakeType: autoblks_shared:autoblkLongitudinalWheel:blkCmb_BrakeType_c1 | autoblks_shared:autoblkLongitudinalWheel:blkCmb_BrakeType_c2 | autoblks_shared:autoblkLongitudinalWheel:blkCmb_BrakeType_c3 | autoblks_shared:autoblkLongitudinalWheel:blkCmb_BrakeType_c4
      mask Callback BrakeType: [~]=vehdynicon('vehdynlibtire',gcb,2)
      mask DialogControl BlockOptions Prompt: autoblks_shared:autoblkLongitudinalWheel:blkDlg_BlockOptions
      mask DialogControl SourceOptions Prompt: vdynblks:vehdynLatTire:blkDlg_SourceOptions
      mask DialogControl tireType Prompt: Tire type:
      mask DialogControl paramOverwrite Prompt: vdynblks:vehdynLatTire:blkPrm_paramOverwrite
      mask DialogControl paramOverwrite Callback: [~]=vehdynicon('vehdynlibtire',gcb,6);
      mask DialogControl BrakeType Prompt: Brake type:
      mask DialogControl plySteer Prompt: Include ply/roll steer behavior
      mask DialogControl turnslip Prompt: Include large turn slip effects
      mask DialogControl WheelParams Prompt: vdynblks:vehdynLatTire:blkDlg_WheelParams
      mask DialogControl brakeParamPanel Prompt: autoblks_shared:autoblkLongitudinalWheel:blkDlg_brakeParamPanel
      mask DialogControl GenParams Prompt: autoblks_shared:autoblkLongitudinalWheel:blkDlg_GenParams
      mask DialogControl mu_static Prompt: Static friction coefficient, mu_static []:
      mask DialogControl mu_kinetic Prompt: Kinetic friction coefficient, mu_kinetic []:
      mask DialogControl DiskBrakeParms Prompt: autoblks_shared:autoblkLongitudinalWheel:blkDlg_DiskBrakeParms
      mask DialogControl disk_abore Prompt: Disc brake actuator bore, disk_abore [m]:
      mask DialogControl Rm Prompt: Brake pad mean radius, Rm [m]:
      mask DialogControl num_pads Prompt: Number of brake pads, num_pads []:
      mask DialogControl DrumBrakeParms Prompt: autoblks_shared:autoblkLongitudinalWheel:blkDlg_DrumBrakeParms
      mask DialogControl drum_abore Prompt: Drum brake actuator bore, drum_abore [m]:
      mask DialogControl drum_a Prompt: Shoe pin to drum center distance, drum_a [m]:
      mask DialogControl drum_c Prompt: Shoe pin center to force application point distance, drum_c [m]:
      mask DialogControl drum_r Prompt: Drum internal radius, drum_r [m]:
      mask DialogControl drum_theta1 Prompt: Shoe pin to pad start angle, drum_theta1 [deg]:
      mask DialogControl drum_theta2 Prompt: Shoe pin to pad end angle, drum_theta2 [deg]:
      mask DialogControl MappedBrakeParms Prompt: autoblks_shared:autoblkLongitudinalWheel:blkDlg_MappedBrakeParms
      mask DialogControl brake_p_bpt Prompt: Brake actuator pressure breakpoints, brake_p_bpt [bar]:
      mask DialogControl brake_n_bpt Prompt: Wheel speed breakpoints, brake_n_bpt [rpm]:
      mask DialogControl f_brake_t Prompt: Brake torque map, f_brake_t [Nm]:
      mask DialogControl PlotBrakeTorqueMap Prompt: autoblks_shared:autoblkLongitudinalWheel:blkDlg_PlotBrakeTorqueMap
      mask DialogControl PlotBrakeTorqueMap Callback: [~]=vehdynicon('vehdynlibtire',gcb,3)
      mask DialogControl tireDataPanel Prompt: vdynblks:vehdynLatTire:blkDlg_tireDataPanel
      mask DialogControl tireParamSet Prompt: Tire file or object, tireParamSet []:
      mask DialogControl getFile Prompt: vdynblks:vehdynLatTire:blkPrm_getFile
      mask DialogControl getFile Callback: [~]=vehdynicon('vehdynlibtire',gcb,4)
      mask DialogControl updateMaskVars Prompt: vdynblks:vehdynLatTire:blkPrm_updateMaskVars
      mask DialogControl updateMaskVars Callback: [~]=vehdynicon('vehdynlibtire',gcb,1)
      mask DialogControl tireParamTab Prompt: vdynblks:vehdynLatTire:blkDlg_tireParamTab
      mask DialogControl simParamPannel Prompt: vdynblks:vehdynLatTire:blkDlg_simParamPannel
      mask DialogControl PRESMAX Prompt: Maximum pressure, PRESMAX [Pa]:
      mask DialogControl PRESMIN Prompt: Minimum pressure, PRESMIN [Pa]:
      mask DialogControl FZMAX Prompt: Maximum normal force, FZMAX [N]:
      mask DialogControl FZMIN Prompt: Minimum normal force, FZMIN [N]:
      mask DialogControl VXLOW Prompt: Velocity tolerance used to handle low velocity situations, VXLOW [m/s]:
      mask DialogControl KPUMAX Prompt: Max allowable slip ratio (absolute), KPUMAX []:
      mask DialogControl KPUMIN Prompt: Minimum allowable slip ratio (absolute), KPUMIN []:
      mask DialogControl ALPMAX Prompt: Max allowable slip angle (absolute), ALPMAX [rad]:
      mask DialogControl ALPMIN Prompt: Minimum allowable slip angle (absolute), ALPMIN [rad]:
      mask DialogControl CAMMAX Prompt: Maximum allowable camber angle, CAMMAX [rad]:
      mask DialogControl CAMMIN Prompt: Minimum allowable camber angle, CAMMIN [rad]:
      mask DialogControl LONGVL Prompt: Nominal longitudinal speed, LONGVL [m/s]:
      mask DialogControl wheelParamPannel Prompt: vdynblks:vehdynLatTire:blkDlg_wheelParamPannel
      mask DialogControl omegao Prompt: Initial rotational velocity, omegao [rad/s]:
      mask DialogControl br Prompt: Rotational damping, br [N*m*s/rad]:
      mask DialogControl UNLOADED_RADIUS Prompt: Unloaded radius, UNLOADED_RADIUS [m]:
      mask DialogControl NOMPRES Prompt: Nominal pressure, NOMPRES [Pa]:
      mask DialogControl FNOMIN Prompt: Nominal normal force, FNOMIN [N]:
      mask DialogControl WIDTH Prompt: Wheel width, WIDTH [m]:
      mask DialogControl RIM_RADIUS Prompt: Rim radius, RIM_RADIUS [m]:
      mask DialogControl inertParamPannel Prompt: vdynblks:vehdynLatTire:blkDlg_inertParamPannel
      mask DialogControl MASS Prompt: Wheel mass, MASS [kg]:
      mask DialogControl IYY Prompt: Rotational inertia (rolling axis), IYY [kg*m^2]:
      mask DialogControl GRAVITY Prompt: Gravity, GRAVITY [m/s^2]:
      mask DialogControl vertParamPannel Prompt: vdynblks:vehdynLatTire:blkDlg_vertParamPannel
      mask DialogControl zo Prompt: Initial tire displacement, zo [m]:
      mask DialogControl zdoto Prompt: Initial wheel vertical velocity (wheel fixed frame), zdoto [m/s]:
      mask DialogControl BREFF Prompt: Effective rolling radius at low load stiffness, BREFF []:
      mask DialogControl DREFF Prompt: Effective rolling radius peak value, DREFF []:
      mask DialogControl FREFF Prompt: Effective rolling radius at high load stiffness, FREFF []:
      mask DialogControl Q_RE0 Prompt: Unloaded to nominal rolling radius ratio, Q_RE0 []:
      mask DialogControl Q_V1 Prompt: Radius rotational speed dependence, Q_V1 []:
      mask DialogControl Q_V2 Prompt: Stiffness rotational speed dependence, Q_V2 []:
      mask DialogControl Q_FZ1 Prompt: Linear load change with deflection, Q_FZ1 []:
      mask DialogControl Q_FZ2 Prompt: Quadratic load change with deflection, Q_FZ2 []:
      mask DialogControl Q_FZ3 Prompt: Linear load change with deflection and quadratic camber, Q_FZ3 []:
      mask DialogControl Q_FCX Prompt: Load response to longitudinal force, Q_FCX []:
      mask DialogControl Q_FCY Prompt: Load response to lateral force, Q_FCY []:
      mask DialogControl Q_FCY2 Prompt: Vertical stiffness change due to lateral load dependency on lateral stiffness, Q_FCY2 []:
      mask DialogControl PFZ1 Prompt: Stiffness response to pressure, PFZ1 []:
      mask DialogControl VERTICAL_STIFFNESS Prompt: Vertical tire stiffness, VERTICAL_STIFFNESS [N/m]:
      mask DialogControl VERTICAL_DAMPING Prompt: Vertical tire damping, VERTICAL_DAMPING [N*s/m]:
      mask DialogControl BOTTOM_OFFST Prompt: Rim bottoming out offset, BOTTOM_OFFST [m]:
      mask DialogControl BOTTOM_STIFF Prompt: Bottoming out stiffness, BOTTOM_STIFF [N/m]:
      mask DialogControl structParamPannel Prompt: vdynblks:vehdynLatTire:blkDlg_structParamPannel
      mask DialogControl LONGITUDINAL_STIFFNESS Prompt: Longitudinal stiffness, LONGITUDINAL_STIFFNESS [N/m]:
      mask DialogControl LATERAL_STIFFNESS Prompt: Lateral stiffness, LATERAL_STIFFNESS [N/m]:
      mask DialogControl PCFX1 Prompt: Linear vertical deflection influence on longitudinal stiffness, PCFX1 []:
      mask DialogControl PCFX2 Prompt: Quadratic vertical deflection influence on longitudinal stiffness, PCFX2 []:
      mask DialogControl PCFX3 Prompt: Pressure dependency on longitudinal stiffness, PCFX3 []:
      mask DialogControl PCFY1 Prompt: Linear vertical deflection influence on lateral stiffness, PCFY1 []:
      mask DialogControl PCFY2 Prompt: Quadratic vertical deflection influence on lateral stiffness, PCFY2 []:
      mask DialogControl PCFY3 Prompt: Pressure dependency on longitudinal stiffness, PCFY3 []:
      mask DialogControl contParamPannel Prompt: vdynblks:vehdynLatTire:blkDlg_contParamPannel
      mask DialogControl Q_RA1 Prompt: Contact length square root term, Q_RA1 []:
      mask DialogControl Q_RA2 Prompt: Contact length linear term, Q_RA2 []:
      mask DialogControl Q_RB1 Prompt: Contact width root term, Q_RB1 []:
      mask DialogControl Q_RB2 Prompt: Contact width linear term, Q_RB2 []:
      mask DialogControl longParamPannel Prompt: vdynblks:vehdynLatTire:blkDlg_longParamPannel
      mask DialogControl PCX1 Prompt: Cfx shape factor, PCX1 []:
      mask DialogControl PDX1 Prompt: Longitudinal friction at nominal normal load, PDX1 []:
      mask DialogControl PDX2 Prompt: Frictional variation with load, PDX2 []:
      mask DialogControl PDX3 Prompt: Frictional variation with camber, PDX3 [1/rad^2]:
      mask DialogControl PEX1 Prompt: Longitudinal curvature at nominal normal load, PEX1 []:
      mask DialogControl PEX2 Prompt: Variation of curvature factor with load, PEX2 []:
      mask DialogControl PEX3 Prompt: Variation of curvature factor with square of load, PEX3 []:
      mask DialogControl PEX4 Prompt: Longitudinal curvature factor with slip, PEX4 []:
      mask DialogControl PKX1 Prompt: Longitudinal slip stiffness at nominal normal load, PKX1 []:
      mask DialogControl PKX2 Prompt: Variation of slip stiffness with load, PKX2 []:
      mask DialogControl PKX3 Prompt: Slip stiffness exponent factor, PKX3 []:
      mask DialogControl PHX1 Prompt: Horizontal shift in slip ratio at nominal normal load, PHX1 []:
      mask DialogControl PHX2 Prompt: Variation of horizontal slip ratio with load, PHX2 []:
      mask DialogControl PVX1 Prompt: Vertical shift in load at nominal normal load, PVX1 []:
      mask DialogControl PVX2 Prompt: Variation of vertical shift with load, PVX2 []:
      mask DialogControl PPX1 Prompt: Linear variation of longitudinal slip stiffness with tire pressure, PPX1 []:
      mask DialogControl PPX2 Prompt: Quadratic variation of longitudinal slip stiffness with tire pressure, PPX2 []:
      mask DialogControl PPX3 Prompt: Linear variation of peak longitudinal friction with tire pressure, PPX3 []:
      mask DialogControl PPX4 Prompt: Quadratic variation of peak longitudinal friction with tire pressure, PPX4 []:
      mask DialogControl RBX1 Prompt: Combined slip Fx slope factor reduction, RBX1 []:
      mask DialogControl RBX2 Prompt: Slip ratio Fx slope reduction variation, RBX2 []:
      mask DialogControl RBX3 Prompt: Camber influence on combined slip Fx stiffness, RBX3 []:
      mask DialogControl RCX1 Prompt: Shape factor for combined slip Fx reduction, RCX1 []:
      mask DialogControl REX1 Prompt: Combined Fx curvature factor, REX1 []:
      mask DialogControl REX2 Prompt: Combined Fx curvature factor with load, REX2 []:
      mask DialogControl RHX1 Prompt: Combined slip Fx shift factor reduction, RHX1 []:
      mask DialogControl overParamPannel Prompt: vdynblks:vehdynLatTire:blkDlg_overParamPannel
      mask DialogControl QSX1 Prompt: Vertical shift of overturning moment, QSX1 []:
      mask DialogControl QSX2 Prompt: Overturning moment due to camber, QSX2 []:
      mask DialogControl QSX3 Prompt: Overturning moment due to Fy, QSX3 []:
      mask DialogControl QSX4 Prompt: Mx combined lateral force load and camber, QSX4 []:
      mask DialogControl QSX5 Prompt: Mx load effect due to lateral force and camber, QSX5 []:
      mask DialogControl QSX6 Prompt: Mx load effect due to B-factor, QSX6 []:
      mask DialogControl QSX7 Prompt: Mx due to camber and load, QSX7 []:
      mask DialogControl QSX8 Prompt: Mx due to lateral force and load, QSX8 []:
      mask DialogControl QSX9 Prompt: Mx due to B-factor of lateral force and load, QSX9 []:
      mask DialogControl QSX10 Prompt: Mx due to vertical force and camber, QSX10 []:
      mask DialogControl QSX11 Prompt: Mx due to B-factor of vertical force and camber, QSX11 []:
      mask DialogControl QSX12 Prompt: Mx due to squared camber, QSX12 []:
      mask DialogControl QSX13 Prompt: Mx due to lateral force, QSX13 []:
      mask DialogControl QSX14 Prompt: Mx due to lateral force with camber, QSX14 []:
      mask DialogControl PPMX1 Prompt: Mx due to inflation pressure, PPMX1 []:
      mask DialogControl lateralParamPanel Prompt: vdynblks:vehdynLatTire:blkDlg_lateralParamPanel
      mask DialogControl PCY1 Prompt: Cfy shape factor for lateral force, PCY1 []:
      mask DialogControl PDY1 Prompt: Lateral friction muy, PDY1 []:
      mask DialogControl PDY2 Prompt: Lateral friction variation of muy with load, PDY2 []:
      mask DialogControl PDY3 Prompt: Lateral friction variation of muy with squared camber, PDY3 []:
      mask DialogControl PEY1 Prompt: Efy lateral curvature at nominal force FZNOM, PEY1 []:
      mask DialogControl PEY2 Prompt: Efy curvature variation with load PEY2, PEY2 []:
      mask DialogControl PEY3 Prompt: Efy curvature constant camber dependency, PEY3 []:
      mask DialogControl PEY4 Prompt: Efy curvature variation with camber, PEY4 []:
      mask DialogControl PEY5 Prompt: Efy curvature variation with camber squared, PEY5 []:
      mask DialogControl PKY1 Prompt: Maximum KFy/FZNOM stiffness, PKY1 []:
      mask DialogControl PKY2 Prompt: Load at maximum KFy/FZNOM stiffness, PKY2 []:
      mask DialogControl PKY3 Prompt: KFy/FZNOM stiffness variation with camber, PKY3 []:
      mask DialogControl PKY4 Prompt: KFy curvature, PKY4 []:
      mask DialogControl PKY5 Prompt: Variation of peak stiffness with squared camber, PKY5 []:
      mask DialogControl PKY6 Prompt: Fy camber stiffness factor, PKY6 []:
      mask DialogControl PKY7 Prompt: Camber stiffness vertical load dependency, PKY7 []:
      mask DialogControl PHY1 Prompt: SHY horizontal shift at FZNOM, PHY1 []:
      mask DialogControl PHY2 Prompt: SHY variation with load, PHY2 []:
      mask DialogControl PVY1 Prompt: Svy/Fz vertical shift at FZNOM, PVY1 []:
      mask DialogControl PVY2 Prompt: Svy/Fz variation with load, PVY2 []:
      mask DialogControl PVY3 Prompt: Svy/Fz variation with camber, PVY3 []:
      mask DialogControl PVY4 Prompt: Svy/Fz variation with load and camber, PVY4 []:
      mask DialogControl PPY1 Prompt: Cornering stiffness variation with inflation pressure, PPY1 []:
      mask DialogControl PPY2 Prompt: Cornering stiffness variation with inflation pressure induced nominal load dependency, PPY2 []:
      mask DialogControl PPY3 Prompt: Linear inflation pressure on peak lateral friction, PPY3 []:
      mask DialogControl PPY4 Prompt: Quadratic inflation pressure on peak lateral friction, PPY4 []:
      mask DialogControl PPY5 Prompt: Inflation pressure effect on camber stiffness, PPY5 []:
      mask DialogControl RBY1 Prompt: Combined Fy reduction slope factor, RBY1 []:
      mask DialogControl RBY2 Prompt: Fy slope reduction with slip angle, RBY2 []:
      mask DialogControl RBY3 Prompt: Fy shift reduction with slip angle, RBY3 []:
      mask DialogControl RBY4 Prompt: Fy combined stiffness variation from camber, RBY4 []:
      mask DialogControl RCY1 Prompt: Fy combined reduction shape factor, RCY1 []:
      mask DialogControl REY1 Prompt: Fy combined curvature factor, REY1 []:
      mask DialogControl REY2 Prompt: Fy combined curvature factor with load, REY2 []:
      mask DialogControl RHY1 Prompt: Fy combined reduction shift factor, RHY1 []:
      mask DialogControl RHY2 Prompt: Fy combined reduction shift factor with load, RHY2 []:
      mask DialogControl RVY1 Prompt: Slip ratio side force Svyk/Muy*Fz at FZNOM, RVY1 []:
      mask DialogControl RVY2 Prompt: Side force Svyk/Muy*Fz variation with load, RVY2 []:
      mask DialogControl RVY3 Prompt: Side force Svyk/Muy*Fz variation with camber, RVY3 []:
      mask DialogControl RVY4 Prompt: Side force Svyk/Muy*Fz variation with slip angle, RVY4 []:
      mask DialogControl RVY5 Prompt: Side force Svyk/Muy*Fz variation with slip ratio, RVY5 []:
      mask DialogControl RVY6 Prompt: Side force Svyk/Muy*Fz variation with slip ratio arctangent, RVY6 []:
      mask DialogControl rollParamPanel Prompt: vdynblks:vehdynLatTire:blkDlg_rollParamPanel
      mask DialogControl QSY1 Prompt: Torque resistance coefficient, QSY1 []:
      mask DialogControl QSY2 Prompt: Torque resistance due to Fx, QSY2 []:
      mask DialogControl QSY3 Prompt: Torque resistance due to speed, QSY3 []:
      mask DialogControl QSY4 Prompt: Torque resistance due to speed^4, QSY4 []:
      mask DialogControl QSY5 Prompt: Torque resistance due to square of camber, QSY5 []:
      mask DialogControl QSY6 Prompt: Torque resistance due to square of camber and load, QSY6 []:
      mask DialogControl QSY7 Prompt: Torque resistance due to load, QSY7 []:
      mask DialogControl QSY8 Prompt: Torque resistance due to pressure, QSY8 []:
      mask DialogControl alignParamPanel Prompt: vdynblks:vehdynLatTire:blkDlg_alignParamPanel
      mask DialogControl QBZ1 Prompt: Trail slope factor for trail Bpt at FZNOM, QBZ1 []:
      mask DialogControl QBZ2 Prompt: Bpt slope variation with load, QBZ2 []:
      mask DialogControl QBZ3 Prompt: Bpt slope variation with square of load, QBZ3 []:
      mask DialogControl QBZ4 Prompt: Bpt slope variation with camber, QBZ4 []:
      mask DialogControl QBZ5 Prompt: Bpt slope variation with absolute value of camber, QBZ5 []:
      mask DialogControl QBZ6 Prompt: Bpt slope variation with square of camber, QBZ6 []:
      mask DialogControl QBZ9 Prompt: Br of Mzr slope scaling factor, QBZ9 []:
      mask DialogControl QBZ10 Prompt: Br of Mzr cornering stiffness factor, QBZ10 []:
      mask DialogControl QCZ1 Prompt: Cpt pneumatic trail shape factor, QCZ1 []:
      mask DialogControl QDZ1 Prompt: Dpt peak trail, QDZ1 []:
      mask DialogControl QDZ2 Prompt: Dpt peak trail variation with load, QDZ2 []:
      mask DialogControl QDZ3 Prompt: Dpt peak trail variation with camber, QDZ3 []:
      mask DialogControl QDZ4 Prompt: Dpt peak trail variation with square of camber, QDZ4 []:
      mask DialogControl QDZ6 Prompt: Dmr peak residual torque, QDZ6 []:
      mask DialogControl QDZ7 Prompt: Dmr peak residual torque variation with load, QDZ7 []:
      mask DialogControl QDZ8 Prompt: Dmr peak residual torque variation with camber, QDZ8 []:
      mask DialogControl QDZ9 Prompt: Dmr peak residual torque variation with camber and load, QDZ9 []:
      mask DialogControl QDZ10 Prompt: Dmr peak residual torque variation with square of camber, QDZ10 []:
      mask DialogControl QDZ11 Prompt: Dmr peak residual torque variation with square of load, QDZ11 []:
      mask DialogControl QEZ1 Prompt: Ept trail curvature at FZNOM, QEZ1 []:
      mask DialogControl QEZ2 Prompt: Ept variation with load, QEZ2 []:
      mask DialogControl QEZ3 Prompt: Ept variation with square of load, QEZ3 []:
      mask DialogControl QEZ4 Prompt: Ept variation with sign of alpha-t, QEZ4 []:
      mask DialogControl QEZ5 Prompt: Ept variation with sign of alpha-t and camber, QEZ5 []:
      mask DialogControl QHZ1 Prompt: Sht horizontal trail shift at FZNOM, QHZ1 []:
      mask DialogControl QHZ2 Prompt: Sht variation with load, QHZ2 []:
      mask DialogControl QHZ3 Prompt: Sht variation with camber, QHZ3 []:
      mask DialogControl QHZ4 Prompt: Sht variation with load and camber, QHZ4 []:
      mask DialogControl PPZ1 Prompt: Inflation pressure influence on trail length, PPZ1 []:
      mask DialogControl PPZ2 Prompt: Inflation pressure influence on residual aligning torque, PPZ2 []:
      mask DialogControl SSZ1 Prompt: Nominal value of s/R0: effect of Fx on Mz, SSZ1 []:
      mask DialogControl SSZ2 Prompt: s/R0 variation with lateral to nominal force ratio, SSZ2 []:
      mask DialogControl SSZ3 Prompt: s/R0 variation with camber, SSZ3 []:
      mask DialogControl SSZ4 Prompt: s/R0 variation with camber and load, SSZ4 []:
      mask DialogControl turnParamPanel Prompt: vdynblks:vehdynLatTire:blkDlg_turnParamPanel
      mask DialogControl PDXP1 Prompt: Fx peak reduction due to spin, PDXP1 []:
      mask DialogControl PDXP2 Prompt: Fx peak reduction due to spin with varying load, PDXP2 []:
      mask DialogControl PDXP3 Prompt: Fx peak reduction due to spin with slip ratio, PDXP3 []:
      mask DialogControl PKYP1 Prompt: Cornering stiffness reduction due to spin, PKYP1 []:
      mask DialogControl PDYP1 Prompt: Fy peak reduction due to spin, PDYP1 []:
      mask DialogControl PDYP2 Prompt: Fy peak reduction due to spin with varying load, PDYP2 []:
      mask DialogControl PDYP3 Prompt: Fy peak reduction due to spin with slip angle, PDYP3 []:
      mask DialogControl PDYP4 Prompt: Fy peak reduction due to square root of spin, PDYP4 []:
      mask DialogControl PHYP1 Prompt: Fy vs. slip angle response lateral shift limit, PHYP1 []:
      mask DialogControl PHYP2 Prompt: Fy vs. slip angle response max lateral shift limit, PHYP2 []:
      mask DialogControl PHYP3 Prompt: Fy vs. slip angle response max lateral shift limit with load, PHYP3 []:
      mask DialogControl PHYP4 Prompt: Fy vs. slip angle response lateral shift curvature factor, PHYP4 []:
      mask DialogControl PECP1 Prompt: Camber stiffness reduction due to spin, PECP1 []:
      mask DialogControl PECP2 Prompt: Camber stiffness reduction due to spin with load, PECP2 []:
      mask DialogControl QDTP1 Prompt: Turn slip pneumatic trail reduction factor, QDTP1 []:
      mask DialogControl QCRP1 Prompt: Turn moment for constant turning and zero longitudinal speed, QCRP1 []:
      mask DialogControl QCRP2 Prompt: Turn slip moment increase with spin at 90deg slip angle, QCRP2 []:
      mask DialogControl QBRP1 Prompt: Residual spin torque reduction from side slip, QBRP1 []:
      mask DialogControl QDRP1 Prompt: Turn slip moment peak magnitude, QDRP1 []:
      mask DialogControl QDRP2 Prompt: Turn slip moment curvature, QDRP2 []:
      mask Display:
      | try
      |     IconInfo = vehdynicon('vehdynlibtire',gcb,8);
      | 
      |     image(IconInfo.image, IconInfo.position);
      | 
      |     for i = 1:numel(IconInfo.lconn)
      |         port_label('lconn', i, IconInfo.lconn{i})
      |     end
      | 
      |     for j = 1:numel(IconInfo.rconn)
      |         port_label('rconn', j, IconInfo.rconn{j})
      |     end
      | 
      |     for k = 1:numel(IconInfo.input)
      |         port_label('input', k, IconInfo.input{k})
      |     end
      | 
      |     for m = 1:numel(IconInfo.output)
      |         port_label('output', m, IconInfo.output{m})
      |     end
      | catch
      |     fprintf('2DOF \n Wheel')
      | end
  Scope6 : Scope  NumInputPorts=2
  Signal Specification : SignalSpecification  Unit=1
  Terminator{,1..6} (7 alike) : Terminator
  Wheels : Outport  VectorParamsAs1DForOutWhenUnconnected=off
  tag scope: WhlVx=global
  wires:
  Combined Slip Wheel 2DOF/8(Mz) -> Terminator6/1
  Combined Slip Wheel 2DOF/5(Fz) -> Terminator3/1
  Combined Slip Wheel 2DOF/6(Mx) -> Terminator4/1
  Combined Slip Wheel 2DOF/7(My) -> Terminator5/1
  Combined Slip Wheel 2DOF/4(Fy) -> Terminator2/1
  Combined Slip Wheel 2DOF/3(Fx) -> Terminator1/1
  Combined Slip Wheel 2DOF/2(Omega) -> Terminator/1
  Signal Specification/1 -> Combined Slip Wheel 2DOF/10(ScaleFctrs)
  Vy/1 -> Scope6/2, Combined Slip Wheel 2DOF/4(Vy)
  Vx/1 -> Scope6/1, [WhlVx], Combined Slip Wheel 2DOF/3(Vx)
  lambda/1 -> Signal Specification/1
  Camber/1 -> Combined Slip Wheel 2DOF/5(Camber)
  r/1 -> Combined Slip Wheel 2DOF/6(YawRate)
  Press/1 -> Combined Slip Wheel 2DOF/7(Prs)
  Gnd/1 -> Combined Slip Wheel 2DOF/8(Gnd)
  DriveTorque/1 -> Combined Slip Wheel 2DOF/2(AxlTrq)
  Brake Pressure/1 -> Combined Slip Wheel 2DOF/1(BrkPrs)
  Combined Slip Wheel 2DOF/1(Info) -> Wheels/1
  FzSusp/1 -> Combined Slip Wheel 2DOF/9(Fext)
